simulink model "simulink_manipulator"  (R2020b)
settings: Solver=VariableStepAuto  StartTime=0.0  StopTime=50  RelTol=1e-3
values from neighbouring files (symbols this model uses):
  A = [0 1 0 0 0 0;0 0 0 0 0 0;0 0 0 1 0 0;0 0 0 0 0 0;0 0 0 0 0 1;0 0 0 0 0 0]    [fuelcell_manipulator.m]
  B = [0 0 0;1/(j1+j2+j3) 0 0;0 0 0;0 1/(m2+4*m3) 0; 0 0 0;0 0 1/m3]    [fuelcell_manipulator.m]
  K = [200 200 0 0 0  0;0 0 500 500 0 0;0 0 0 0 600 600]    [fuelcell_manipulator.m]
settings Model: Creator=mori  LastModifiedBy=mori

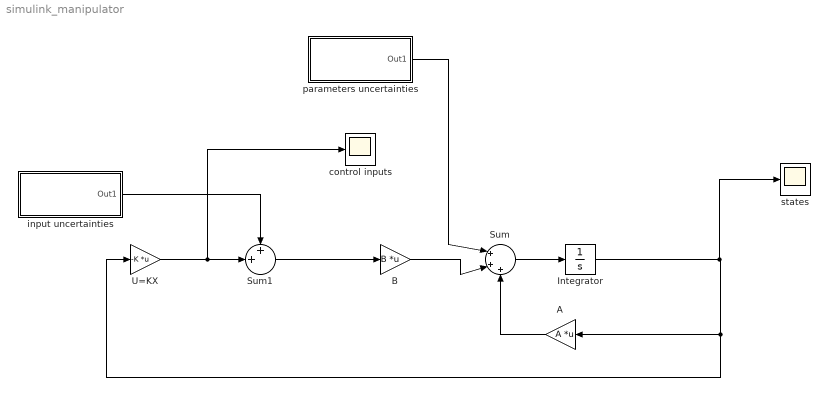
== system simulink_manipulator ==
  " parameters uncertainties" : Subsystem
  A : Gain  Gain=A  Multiplication=Matrix(K*u) (u vector)
  B : Gain  Gain=B  Multiplication=Matrix(K*u) (u vector)
  Integrator : Integrator  InitialCondition=[5,5,5,5,5,5]
  Sum : Sum  Inputs=|+++
  Sum1 : Sum  Inputs=++|
  U=KX : Gain  Gain=-K  Multiplication=Matrix(K*u) (u vector)
  control inputs : Scope
  input uncertainties : Subsystem
  states : Scope
  wires:
  input uncertainties/1(Out1) -> Sum1/1
  B/1 -> Sum/2
  A/1 -> Sum/3
  Integrator/1 -> A/1, U=KX/1, states/1
  Sum/1 -> Integrator/1
  " parameters uncertainties"/1(Out1) -> Sum/1
  U=KX/1 -> control inputs/1, Sum1/2
  Sum1/1 -> B/1

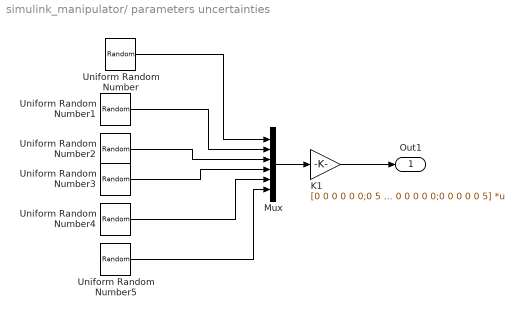
== system simulink_manipulator/ parameters uncertainties ==
  K1 : Gain  Gain="[0 0 0 0 0 0;0 5 0  0 0 0;0 0 0 0 0 0;0 0 0 5 0 0;0 0 0 0 0 0;0 0 0 0 0 5]"  Multiplication=Matrix(K*u) (u vector)
  Mux : Mux  Inputs=6
  Uniform Random Number{,1..5} (6 alike) : UniformRandomNumber  SampleTime=0.1
  Out1 : Outport
  wires:
  K1/1 -> Out1/1
  Mux/1 -> K1/1
  Uniform Random Number1/1 -> Mux/2
  Uniform Random Number2/1 -> Mux/3
  Uniform Random Number/1 -> Mux/1
  Uniform Random Number3/1 -> Mux/4
  Uniform Random Number4/1 -> Mux/5
  Uniform Random Number5/1 -> Mux/6

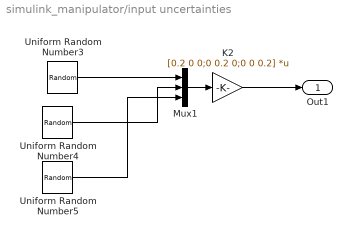
== system simulink_manipulator/input uncertainties ==
  K2 : Gain  Gain=[0.2 0 0;0 0.2 0;0 0 0.2]  Multiplication=Matrix(K*u) (u vector)
  Mux1 : Mux  Inputs=3
  Uniform Random Number3 : UniformRandomNumber  SampleTime=0.1
  Uniform Random Number4 : UniformRandomNumber  SampleTime=0.1
  Uniform Random Number5 : UniformRandomNumber  SampleTime=0.1
  Out1 : Outport
  wires:
  K2/1 -> Out1/1
  Uniform Random Number3/1 -> Mux1/1
  Mux1/1 -> K2/1
  Uniform Random Number4/1 -> Mux1/2
  Uniform Random Number5/1 -> Mux1/3
